simulink model "LinPredict"  (Simulink 7.7)
settings: Solver=FixedStepDiscrete  StartTime=0.0  StopTime=5000  RelTol=1e-3
values from neighbouring files (symbols this model uses):
  D = [  1 -1  1 -1  1  1 -1 -1 ... (first row only)    [cdma.m]    (also in compressed_sampling.m = idct(eye(5000,5000)))
libraries: simulink x1, dspadpt3 x1, dspsrcs4 x1
settings Model: Creator=Arun  LastModifiedBy=ArunKB

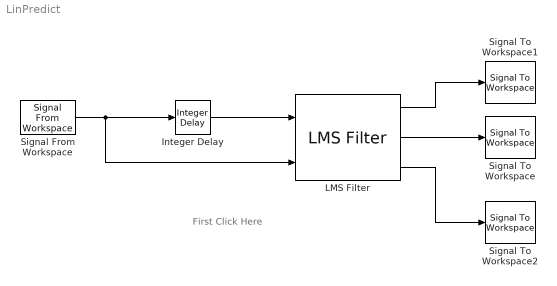
== system LinPredict ==
  note: First Click Here
  Integer Delay : simulink/Discrete/Integer Delay  NumDelays=1  vinit=0.0  samptime=-1
  LMS Filter : dspadpt3/LMS Filter  Algo=LMS  L=17  stepflag=Dialog  mu=.01  leakage=1.0  ic=0  Adapt=off  resetflag=None  weights=on  secondCoeffMode=User-defined  secondCoeffWordLength=2  secondCoeffFracLength=15  accum2Mode=User-defined  accum2FracLength=20  prodOutput2Mode=User-defined  prodOutput2FracLength=20  prodOutput3Mode=User-defined  prodOutput3FracLength=20  prodOutput4Mode=User-defined  prodOutput4FracLength=20  quotientMode=User-defined  quotientFracLength=20  roundingMode=Floor  overflowMode=off  addnparflag=off
  Signal From Workspace : dspsrcs4/Signal From Workspace  SystemSampleTime=-1  X=n  Ts=1  nsamps=1  OutputAfterFinalValue=Setting to zero  ignoreOrWarnInputAndFrameLengths=off
  Signal To Workspace : SignalToWorkspace  VariableName=error  SaveFormat=Array  Save2DMode=2-D array (concatenate along first dimension)
      settings: CopyFcn=dspblkcopystw(gcbh);
  Signal To Workspace1 : SignalToWorkspace  VariableName=output  SaveFormat=Array  Save2DMode=2-D array (concatenate along first dimension)
      settings: CopyFcn=dspblkcopystw(gcbh);
  Signal To Workspace2 : SignalToWorkspace  VariableName=wts  SaveFormat=Array  Save2DMode=2-D array (concatenate along first dimension)
      settings: CopyFcn=dspblkcopystw(gcbh);  MaxDataPoints=17
  wires:
  Integer Delay/1 -> LMS Filter/1
  Signal From Workspace/1 -> Integer Delay/1, LMS Filter/2
  LMS Filter/2 -> Signal To Workspace/1
  LMS Filter/1 -> Signal To Workspace1/1
  LMS Filter/3 -> Signal To Workspace2/1
